simulink model "December_1_Simulink"  (R2023a)
settings: Solver=VariableStepAuto  StartTime=0.0  StopTime=10.0  RelTol=1e-3
model workspace (MAT data in the model file):
  Voice_or_File = 0
undefined symbols (not defined in the file): fdesignblkfcn, gcbh
libraries: audiofilters x4, dspfdesign x3, dspsigops x3, dspsnks4 x1, dspmlti4 x1, dspxfrm3 x1, dspvision x1, audiomeasurements x1
settings Model: Creator=hunte  LastModifiedBy=hunte

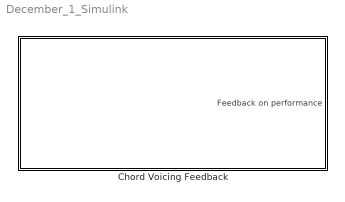
== system December_1_Simulink ==
  "Chord Voicing Feedback " : Subsystem

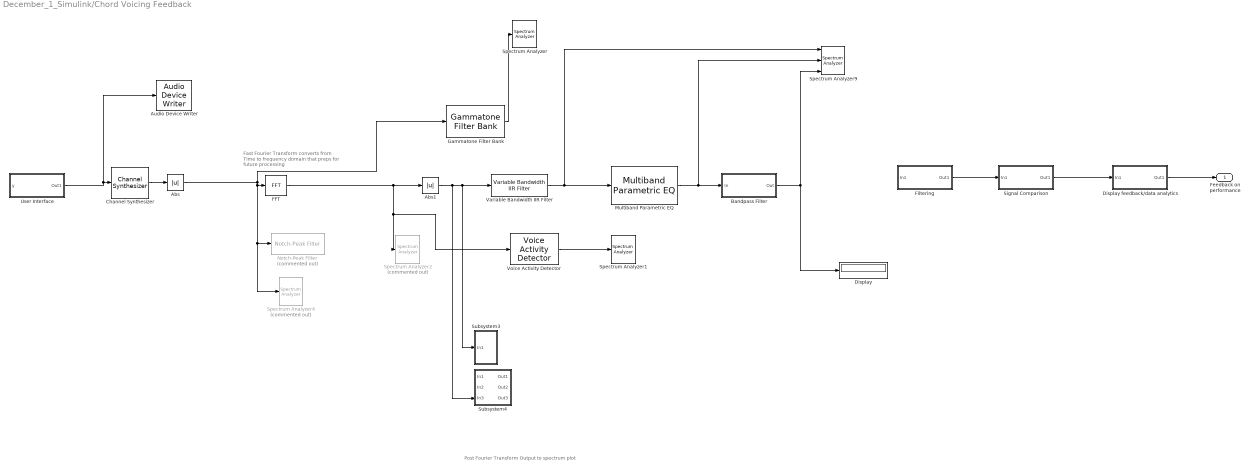
== system December_1_Simulink/Chord Voicing Feedback  ==
  note: Fast Fourier Transform converts from Time to frequency domain that preps for future processing
  note: Post Fourier Transform Output to spectrum plot
  Abs : Abs  SaturateOnIntegerOverflow=off
  Abs1 : Abs  SaturateOnIntegerOverflow=off
  Audio Device Writer : dspsnks4/Audio Device Writer  Driver=DirectSound  Device=Default  InheritSampleRate=on  SampleRate=44100  BitDepth=16-bit integer  BufferSize=4096  NumBuffers=10  DefaultOutputChannelMapping=on  OutputChannelMapping=1:2  OutputNumUnderrunSamples=off  DriverIdx=1  DeviceWarnFlag=''
  Bandpass Filter : Subsystem  DialogController=fdesignblkfcn  InitFcn=fdesignblkfcn(gcbh, {'InitFcn'});  mask(Bandpass Filter){}
      mask help: dsp:DSPFilterDesignBlockDialog:BandpassFdesign_MaskDesc
      settings: CopyFcn=fdesignblkfcn(gcbh, {'CopyFcn'});
      mask Help: helpview(mapfilelocation('dsp'), 'dspbandpassfilter');
      mask Display: disp('Bandpass');
  Channel Synthesizer : dspmlti4/Channel Synthesizer  Specification=Number of taps per band and stopband attenuation  CoefficientsPort=off  NumTapsPerBand=100  StopbandAttenuation=20  LowpassCoefficients=rcosdesign( 0.25, 6, 8, 'sqrt' )  SimulateUsing=Interpreted execution
  Display : Display
  Display feedback/data analytics : Subsystem
  FFT : dspxfrm3/FFT  FFTImplementation=Auto  CompMethod=Table lookup  TableOpt=NEW  TableOptActive=Speed  BitRevOrder=off  Normalize=off  InheritFFTLength=on  FFTLength=64  WrapInput=on  roundingMode=Floor  overflowMode=off  firstCoeffDataTypeStr=Inherit: Same word length as input  firstCoeffLastDataTypeStr=Inherit: Same word length as input  outputMin=[]  outputMax=[]
  Filtering : Subsystem
  Gammatone Filter Bank : audiofilters/Gammatone Filter Bank  FrequencyRange=[50 8000]  NumFilters=32  InheritSampleRate=off  SampleRate=16000  BandsAsSeparateOutputPorts=off  WorkspaceVariableName=myFilt  OverwriteExportVariable=on  SimulateUsing=Interpreted execution
      settings: LibrarySourceBlock=audiofeatures/Gammatone Filter Bank
  Multiband Parametric EQ : audiofilters/Multiband Parametric EQ  EQOrder=2  NumEQBands=3  FrequenciesPort=off  Frequencies=[100 181 325]  PeakGainsPort=off  PeakGains=[20 20 20]  QualityFactorsPort=off  QualityFactors=[1.6 1.6 1.6]  InheritSampleRate=off  SampleRate=44100  WorkspaceVariableName=myFilt  OverwriteExportVariable=on  HasLowShelfFilter=off  LowShelfCutoffPort=off  LowShelfCutoff=200  LowShelfSlopePort=off  LowShelfSlope=1.5  LowShelfGainPort=off  LowShelfGain=0  HasHighShelfFilter=off  HighShelfCutoffPort=off  HighShelfCutoff=15e3  HighShelfSlopePort=off  HighShelfSlope=1.5  HighShelfGainPort=off  HighShelfGain=0  HasLowpassFilter=off  LowpassCutoffPort=off  LowpassCutoff=18e3  LowpassSlopePort=off  LowpassSlope=12  HasHighpassFilter=off  HighpassCutoffPort=off  HighpassCutoff=20  HighpassSlopePort=off  HighpassSlope=30  Oversample=off  SimulateUsing=Code generation
  Notch-Peak Filter : dspfdesign/Notch-Peak Filter  Commented=on  Specification=Bandwidth and center frequency  BandwidthPort=off  Bandwidth=2205  QualityFactorPort=off  QualityFactor=5  CenterFrequencyPort=off  CenterFrequency=11025  BandwidthCoefficientPort=off  BandwidthCoefficient=0.72654  CenterFrequencyCoefficientPort=off  CenterFrequencyCoefficient=0  Output=Notch and Peak  InheritSampleRate=off  SampleRate=44100  SimulateUsing=Code generation
  Signal Comparison : Subsystem
  Spectrum Analyzer : SpectrumAnalyzer  WindowPosition=[697.000000,588.000000,800.000000,500.000000,]  ScopeFrameLocation=window  SampleRateSource=Property  SampleRate=44.1e3  PlotAsTwoSidedSpectrum=off  FrequencyScale=Log  FrequencySpan=Start and stop frequencies  StartFrequency=20  StopFrequency=20e3  YLimits=[-254.97779991,42.98478397]  ColorLimits=[-20 80]  ShowLegend=on  DefaultConfigurationName=spbscopes.SpectrumAnalyzerBlockCfg  IsFrequencyInputMode=0  FrequencyVectorPort=0  FrequencyVectorFromPort=0  FrequencyInputRBWPort=0  FrequencyInputRBWFromPort=0
  Spectrum Analyzer1 : SpectrumAnalyzer  WindowPosition=[880.000000,470.000000,800.000000,500.000000,]  ScopeFrameLocation=window  SampleRateSource=Property  SampleRate=44.1e3  PlotAsTwoSidedSpectrum=off  FrequencyScale=Log  FrequencySpan=Start and stop frequencies  StartFrequency=20  StopFrequency=20e3  YLimits=[-20 80]  ColorLimits=[-20 80]  DefaultConfigurationName=spbscopes.SpectrumAnalyzerBlockCfg  IsFrequencyInputMode=0  FrequencyVectorPort=0  FrequencyVectorFromPort=0  FrequencyInputRBWPort=0  FrequencyInputRBWFromPort=0
  Spectrum Analyzer2 : SpectrumAnalyzer  Commented=on  WindowPosition=[880.000000,118.000000,800.000000,500.000000,]  ScopeFrameLocation=window  SampleRateSource=Property  SampleRate=44.1e3  PlotAsTwoSidedSpectrum=off  FrequencyScale=Log  FrequencySpan=Start and stop frequencies  StartFrequency=20  StopFrequency=20e3  YLimits=[-60.46925282,-35.33646028]  ColorLimits=[-20 80]  ShowLegend=on  DefaultConfigurationName=spbscopes.SpectrumAnalyzerBlockCfg  IsFrequencyInputMode=0  FrequencyVectorPort=0  FrequencyVectorFromPort=0  FrequencyInputRBWPort=0  FrequencyInputRBWFromPort=0
  Spectrum Analyzer4 : SpectrumAnalyzer  Commented=on  WindowPosition=[2.000000,50.000000,1021.000000,987.000000,]  ScopeFrameLocation=window  SampleRateSource=Property  SampleRate=44.1e3  PlotAsTwoSidedSpectrum=off  FrequencyScale=Log  FrequencySpan=Start and stop frequencies  StartFrequency=20  StopFrequency=20e3  YLimits=[-118.99638748,24.61030048]  ColorLimits=[-20 80]  SelectedToolstripTab=spectrumAnalyzerToolstrip.measurementsTab  DefaultConfigurationName=spbscopes.SpectrumAnalyzerBlockCfg  IsFrequencyInputMode=0  FrequencyVectorPort=0  FrequencyVectorFromPort=0  FrequencyInputRBWPort=0  FrequencyInputRBWFromPort=0
  Spectrum Analyzer9 : SpectrumAnalyzer  NumInputPorts=3  WindowPosition=[1.000000,49.000000,1707.000000,996.000000,]  ScopeFrameLocation=window  SampleRateSource=Property  SampleRate=44.1e3  PlotAsTwoSidedSpectrum=off  FrequencyScale=Log  FrequencySpan=Start and stop frequencies  StartFrequency=20  StopFrequency=20e3  YLimits=[-185.76195608,83.01703193]  ColorLimits=[-20 80]  ShowLegend=on  SelectedToolstripTab=spectrumAnalyzerToolstrip.measurementsTab  DefaultConfigurationName=spbscopes.SpectrumAnalyzerBlockCfg  IsFrequencyInputMode=0  FrequencyVectorPort=0  FrequencyVectorFromPort=0  FrequencyInputRBWPort=0  FrequencyInputRBWFromPort=0
  Subsystem3 : Subsystem
  Subsystem4 : Subsystem
  User Interface : Subsystem
  Variable Bandwidth IIR Filter : dspfdesign/Variable Bandwidth IIR Filter  FilterType=Bandpass  FilterOrder=32  PassbandFrequencyPort=off  PassbandFrequency=512  CenterFrequencyPort=off  CenterFrequency=369.994  BandwidthPort=off  Bandwidth=261.624  PassbandRipple=1  StopbandAttenuation=60  SampleRateMode=Specify on dialog  SampleRate=44100  SimulateUsing=Code generation
  Voice Activity Detector : audiomeasurements/Voice Activity Detector  InputDomain=Frequency  Window=Hann  SidelobeAttenuation=60  InheritFFTLength=on  FFTLength=1024  SilenceToSpeechProbabilityPort=off  SilenceToSpeechProbability=0.2  SpeechToSilenceProbabilityPort=off  SpeechToSilenceProbability=0.1  OutputNoiseVariance=off  SimulateUsing=Code generation
  Feedback on performance : Outport
  wires:
  FFT/1 -> Spectrum Analyzer2/1, Voice Activity Detector/1, Abs1/1
  Display feedback/data analytics/1(Out1) -> Feedback on performance/1
  Filtering/1(Out1) -> Signal Comparison/1(In1)
  Signal Comparison/1(Out1) -> Display feedback/data analytics/1(In1)
  User Interface/1(Out1) -> Channel Synthesizer/1, Audio Device Writer/1
  Abs/1 -> Gammatone Filter Bank/1, Spectrum Analyzer4/1, Notch-Peak Filter/1, FFT/1
  Abs1/1 -> Subsystem3/1(In1), Variable Bandwidth IIR Filter/1, Subsystem4/3(In3)
  Multiband Parametric EQ/1 -> Bandpass Filter/1(In), Spectrum Analyzer9/2
  Bandpass Filter/1(Out) -> Display/1, Spectrum Analyzer9/3
  Variable Bandwidth IIR Filter/1 -> Spectrum Analyzer9/1, Multiband Parametric EQ/1
  Gammatone Filter Bank/1 -> Spectrum Analyzer/1
  Channel Synthesizer/1 -> Abs/1
  Voice Activity Detector/1 -> Spectrum Analyzer1/1

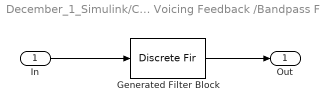
== system December_1_Simulink/Chord Voicing Feedback /Bandpass Filter ==
  In : Inport
  Generated Filter Block : DiscreteFir  Tag=BlockMethodSubSystem  Coefficients=[-0.0008992291487744296 0.0016414518747943749 0.0031352071842225397 -0.0040707550828814922 -0.0063731852227904111 0.0074874286806090491 0.0098354319566295711 -0.010189316513446216 -0.011302794465874122 0.0096929185841818435 0.0079428653987464216 -0.0031368247881221642 0.0028299878877943137 -0.011508674243001471 -0.022080136219461581 0.034245325424507672 0.048356661648905473 -0.062355369169884239 -0.077503478162593897 0.090687768153125653 0.10353171105844157 -0.11297860084229834 -0.12035866024978455 0.12379360801539134 0.12379360801539134 -0.12035866024978455 -0.11297860084229834 0.10353171105844157 0.090687768153125653 -0.077503478162593897 -0.062355369169884239 0.048356661648905473 0.034245325424507672 -0.022080136219461581 -0.011508674243001471 0.0028299878877943137 -0.0031368247881221642 0.0079428653987464216 0.0096929185841818435 -0.011302794465874122 -0.010189316513446216 0.0098354319566295711 0.0074874286806090491 -0.0063731852227904111 -0.0040707550828814922 0.0031352071842225397 0.0016414518747943749 -0.0008992291487744296]  InputProcessing=Columns as channels (frame based)
  Out : Outport  VectorParamsAs1DForOutWhenUnconnected=off
  wires:
  In/1 -> Generated Filter Block/1
  Generated Filter Block/1 -> Out/1

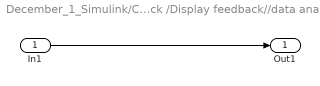
== system December_1_Simulink/Chord Voicing Feedback /Display feedback//data analytics ==
  In1 : Inport
  Out1 : Outport
  wires:
  In1/1 -> Out1/1

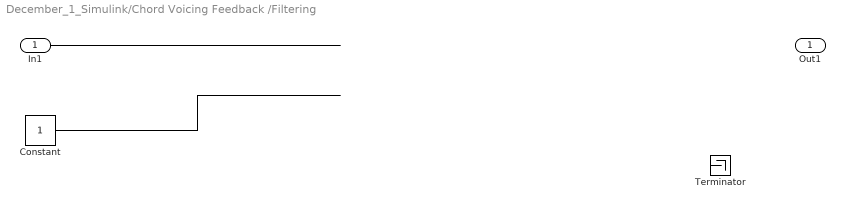
== system December_1_Simulink/Chord Voicing Feedback /Filtering ==
  In1 : Inport
  Constant : Constant
  Terminator : Terminator
  Out1 : Outport
  wires:
  In1/1 -> ?
  ? -> Terminator/1
  Constant/1 -> ?

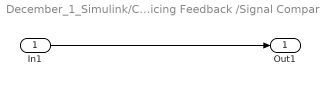
== system December_1_Simulink/Chord Voicing Feedback /Signal Comparison ==
  In1 : Inport
  Out1 : Outport
  wires:
  In1/1 -> Out1/1

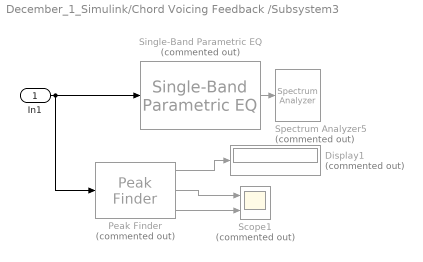
== system December_1_Simulink/Chord Voicing Feedback /Subsystem3 ==
  In1 : Inport
  Display1 : Display  Commented=on
  Peak Finder : dspsigops/Peak Finder  Commented=on  polarity=Maxima and Minima  indexBase=Zero  outputIdx=on  outputVal=off  maxPeaks=99  NoiseDistinguish=off  thresh=0  roundingMode=Floor  overflowMode=off
      settings: allowOverrides=off
  Scope1 : Scope  Commented=on  NumInputPorts=2
  Single-Band Parametric EQ : audiofilters/Single-Band Parametric EQ  Commented=on  FilterOrder=2  Specification=Bandwidth and center frequency  CenterFrequencyPort=off  CenterFrequency=3626  BandwidthPort=off  Bandwidth=7200  QualityFactorPort=off  QualityFactor=5  PeakGaindBPort=off  PeakGaindB=27.0  InheritSampleRate=off  SampleRate=44100  SimulateUsing=Interpreted execution
  Spectrum Analyzer5 : SpectrumAnalyzer  Commented=on  WindowPosition=[204.000000,-124.000000,800.000000,500.000000,]  ScopeFrameLocation=window  SampleRateSource=Property  SampleRate=44.1e3  PlotAsTwoSidedSpectrum=off  FrequencyScale=Log  FrequencySpan=Start and stop frequencies  StartFrequency=20  StopFrequency=20e3  YLimits=[-16.66753513,61.72710433]  ColorLimits=[-20 80]  DefaultConfigurationName=spbscopes.SpectrumAnalyzerBlockCfg  IsFrequencyInputMode=0  FrequencyVectorPort=0  FrequencyVectorFromPort=0  FrequencyInputRBWPort=0  FrequencyInputRBWFromPort=0
  wires:
  Peak Finder/1 -> Display1/1
  Peak Finder/3 -> Scope1/2
  Peak Finder/2 -> Scope1/1
  Single-Band Parametric EQ/1 -> Spectrum Analyzer5/1
  In1/1 -> Single-Band Parametric EQ/1, Peak Finder/1

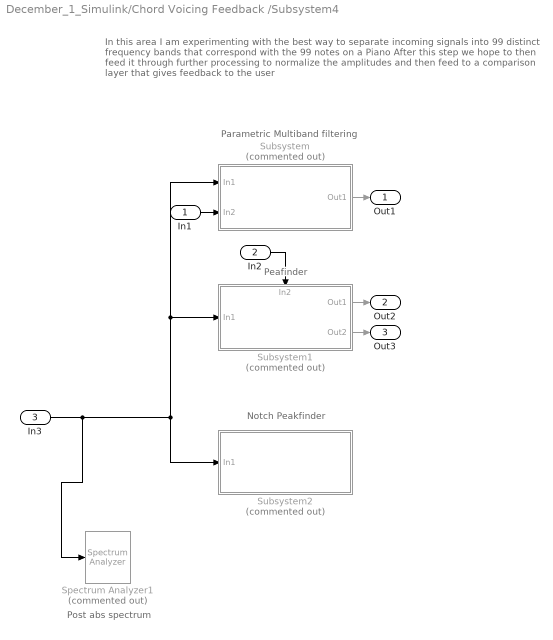
== system December_1_Simulink/Chord Voicing Feedback /Subsystem4 ==
  note: In this area I am experimenting with the best way to separate incoming signals into 99 distinct frequency bands that correspond with the 99 notes on a Piano
      |
      | After this step we hope to then feed it through further processing to normalize the amplitudes and then feed to a comparison layer that gives feedback to the user
  note: Notch Peakfinder
  note: Peafinder
  note: Parametric Multiband filtering
  note: Post abs spectrum
  In1 : Inport
  In2 : Inport  Port=2
  In3 : Inport  Port=3
  Spectrum Analyzer1 : SpectrumAnalyzer  Commented=on  WindowPosition=[160.000000,424.000000,800.000000,500.000000,]  ScopeFrameLocation=window  SampleRateSource=Property  SampleRate=44.1e3  PlotAsTwoSidedSpectrum=off  FrequencyScale=Log  FrequencySpan=Start and stop frequencies  StartFrequency=20  StopFrequency=20e3  YLimits=[-73.0740934,-18.63514495]  ColorLimits=[-20 80]  ShowLegend=on  DefaultConfigurationName=spbscopes.SpectrumAnalyzerBlockCfg  IsFrequencyInputMode=0  FrequencyVectorPort=0  FrequencyVectorFromPort=0  FrequencyInputRBWPort=0  FrequencyInputRBWFromPort=0
  Subsystem : Subsystem  Commented=on
  Subsystem1 : Subsystem  Commented=on
      settings: PortSchema="{\"entries\":[{\"content\":{\"sides\":[{\"content\":{\"connectorIds\":[\"In1\"]},\"type\":\"ConnectorPlacement.EquallySpacedRectSide\",\"uuid\":\"1f4cc2a7-45a5-4ee2-bbe2-5009f707d4e1\"},{\"content\":{\"connectorIds\":[\"Out1\",\"Out2\"],\"side\":\"RIGHT\"},\"type\":\"ConnectorPlacement.EquallySpacedRectSide\",\"uuid\":\"c41a11ba-159e-4698-b840-837f180e5a46\"},{\"content\":{\"connectorIds\":[\"In2\"],\"side\":\"TOP\"},\"type\":\"ConnectorPlacement.EquallySpacedRectSide\",\"uuid\":\"6f77a8f9-ed6e-468a-8709-2f3e2c302975\"}]},\"type\":\"ConnectorPlacement.EquallySpacedConnector\",\"uuid\":\"1c181e66-6eec-4944-a04a-d6183d1ae9d9\"}],\"packageUris\":[\"http://schema.mathworks.com/mf0/Connector/R2020b\"],\"version\":\"1.0\"}"
  Subsystem2 : Subsystem  Commented=on
  Out1 : Outport
  Out2 : Outport  Port=2
  Out3 : Outport  Port=3
  wires:
  In3/1 -> Spectrum Analyzer1/1, Subsystem2/1(In1), Subsystem/1(In1), Subsystem1/1(In1)
  In2/1 -> Subsystem1/2(In2)
  In1/1 -> Subsystem/2(In2)
  Subsystem1/2(Out2) -> Out3/1
  Subsystem/1(Out1) -> Out1/1
  Subsystem1/1(Out1) -> Out2/1

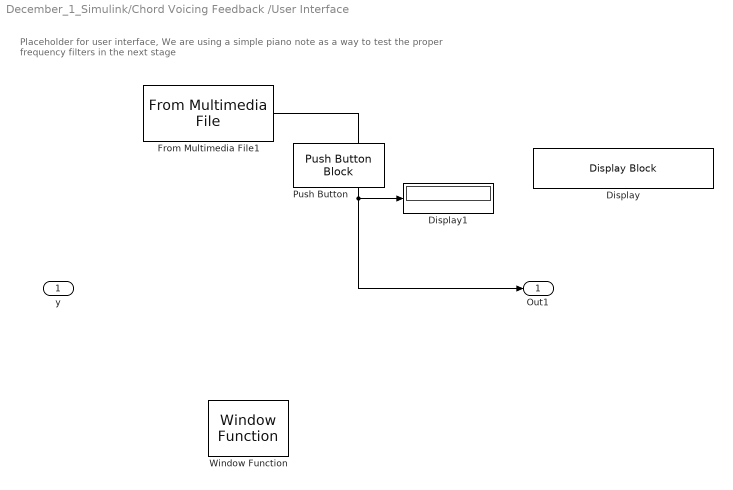
== system December_1_Simulink/Chord Voicing Feedback /User Interface ==
  note: Placeholder for user interface, We are using a simple piano note as a way to test the proper frequency filters in the next stage
  y : Inport
  Display : DisplayBlock  LabelPosition=Hide  Transparency=1
  Display1 : Display
      settings: Format=bank
  From Multimedia File1 : dspvision/From Multimedia File  inputFilename=C:\Users\hunte\Downloads\Cmajor.mp3  readRange=[1 Inf]  loop=on  numPlays=inf  outputStreams=Audio only  videoDataType=single  audioDataType=double  inheritSampleTime=on  userDefinedSampleTime=1/30  noAudioOutput=off  isIntensityVideo=off  fourcc=RGB  colorVideoFormat=Separate color signals  outputEOF=off  dataOrg=Column-major  audioFrameSize=1024  computeAudioFrameSize=off  outSamplingMode=Sample based
      settings: LibrarySourceBlock=audiosources/From Multimedia File
  Push Button : PushButtonBlock
  Window Function : dspsigops/Window Function  winmode=Apply window to input  wintype=Boxcar  sampmode=Discrete  samptime=1  N=64  Rs=50  beta=10  winsamp=Periodic  UserWindow=hamming  OptParams=off  UserParams={'symmetric'}  dataType=double  isSigned=on  wordLen=16  udDataType=sfix(16)  fracBitsMode=Best precision  numFracBits=15  roundingMode=Floor  overflowMode=off  numSidelobes=4  sidelobeLevel=-30
  Out1 : Outport
  wires:
  From Multimedia File1/1 -> Out1/1, Display1/1

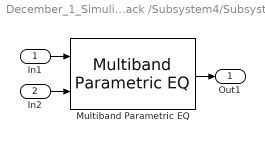
== system December_1_Simulink/Chord Voicing Feedback /Subsystem4/Subsystem ==
  In1 : Inport
  In2 : Inport  Port=2
  Multiband Parametric EQ : audiofilters/Multiband Parametric EQ  EQOrder=10  NumEQBands=10  FrequenciesPort=on  Frequencies=[100 181 325]  PeakGainsPort=off  PeakGains=[0 0 0 0 0 0 0 0 0 0]  QualityFactorsPort=off  QualityFactors=[1.6 1.6 1.6 1.6 1.6 1.6 1.6 1.6 1.6 1.6]  InheritSampleRate=off  SampleRate=44100  WorkspaceVariableName=myFilt  OverwriteExportVariable=on  HasLowShelfFilter=off  LowShelfCutoffPort=off  LowShelfCutoff=200  LowShelfSlopePort=off  LowShelfSlope=1.5  LowShelfGainPort=off  LowShelfGain=0  HasHighShelfFilter=off  HighShelfCutoffPort=off  HighShelfCutoff=15e3  HighShelfSlopePort=off  HighShelfSlope=1.5  HighShelfGainPort=off  HighShelfGain=0  HasLowpassFilter=off  LowpassCutoffPort=off  LowpassCutoff=18e3  LowpassSlopePort=off  LowpassSlope=12  HasHighpassFilter=off  HighpassCutoffPort=off  HighpassCutoff=20  HighpassSlopePort=off  HighpassSlope=30  Oversample=off  SimulateUsing=Code generation
  Out1 : Outport
  wires:
  In2/1 -> Multiband Parametric EQ/2
  Multiband Parametric EQ/1 -> Out1/1
  In1/1 -> Multiband Parametric EQ/1

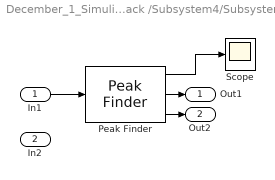
== system December_1_Simulink/Chord Voicing Feedback /Subsystem4/Subsystem1 ==
  In1 : Inport
  In2 : Inport  Port=2
  Peak Finder : dspsigops/Peak Finder  polarity=Maxima  indexBase=Zero  outputIdx=on  outputVal=on  maxPeaks=3  NoiseDistinguish=off  thresh=0  roundingMode=Floor  overflowMode=off
      settings: allowOverrides=off
  Scope : Scope
  Out1 : Outport
  Out2 : Outport  Port=2
  wires:
  Peak Finder/1 -> Scope/1
  In1/1 -> Peak Finder/1
  Peak Finder/3 -> Out2/1
  Peak Finder/2 -> Out1/1

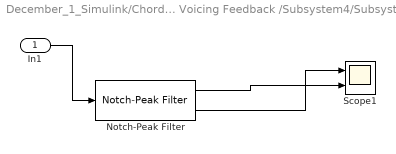
== system December_1_Simulink/Chord Voicing Feedback /Subsystem4/Subsystem2 ==
  In1 : Inport
  Notch-Peak Filter : dspfdesign/Notch-Peak Filter  Specification=Bandwidth and center frequency  BandwidthPort=off  Bandwidth=2205  QualityFactorPort=off  QualityFactor=5  CenterFrequencyPort=off  CenterFrequency=11025  BandwidthCoefficientPort=off  BandwidthCoefficient=0.72654  CenterFrequencyCoefficientPort=off  CenterFrequencyCoefficient=0  Output=Notch and Peak  InheritSampleRate=off  SampleRate=44100  SimulateUsing=Code generation
  Scope1 : Scope  NumInputPorts=2
  wires:
  Notch-Peak Filter/2 -> Scope1/1
  Notch-Peak Filter/1 -> Scope1/2
  In1/1 -> Notch-Peak Filter/1
